simulink model "DemoControlSys"  (R2022b)
settings: Solver=VariableStepAuto  StartTime=0.0  StopTime=10.0  RelTol=1e-3
undefined symbols (not defined in the file): k, ka, kd, ki, kp, kpos, kv
settings Model: Creator=Ilya_Andriyanov  LastModifiedBy=Ilya_Andriyanov

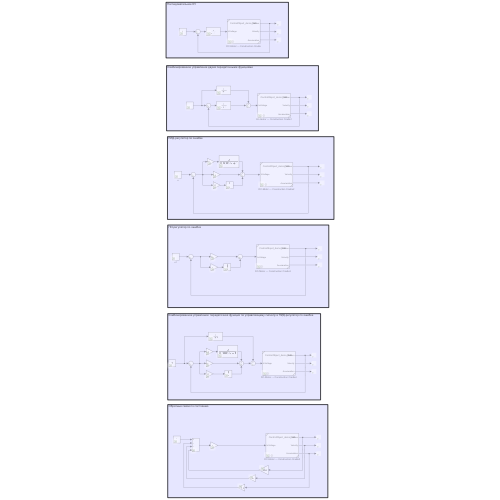
[thumbnail: Simulink's stored preview of the top-level diagram]
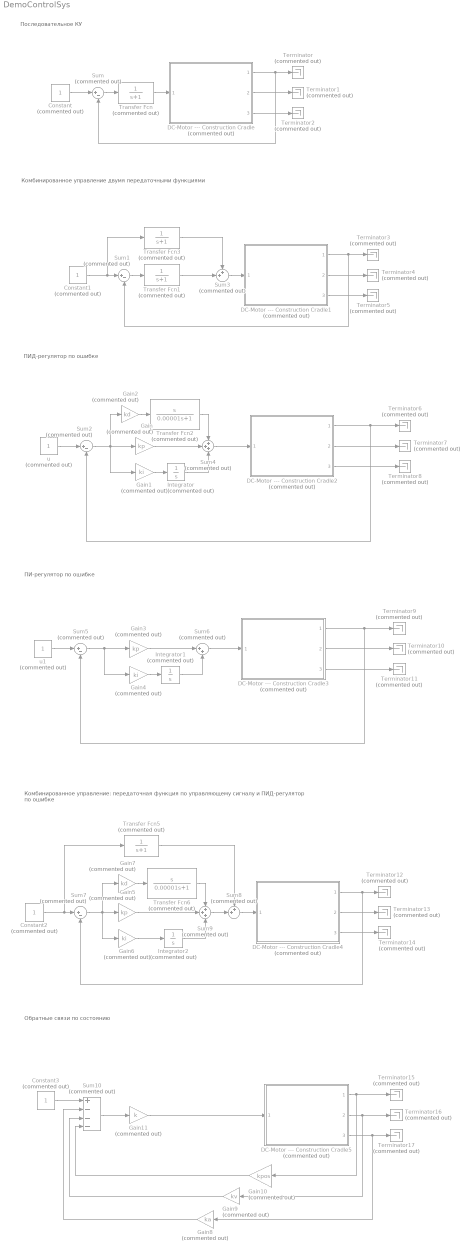
== system DemoControlSys ==
  note: Обратные связи по состоянию
  note: Комбинированное управление: передаточная функция по управляющему сигналу и ПИД-регулятор по ошибке
  note: ПИ-регулятор по ошибке
  note: ПИД-регулятор по ошибке
  note: Комбинированное управление двумя передаточными функциями
  note: Последовательное КУ
  Constant{,1..3} (4 alike) : Constant  Commented=on
  DC-Motor --- Construction Cradle{,1..5} (6 alike) : Subsystem  Commented=on  ReferencedSubsystem=ControlObject_demo_22b  L=0.1  R=0.2  km=1e-3  kw=0.2  J_motor=1e-6  vis_friction_coef_motor=0.001  i_gear=100  J_gear=0.001  vis_friction_coef_gear=0.001  r_wheel=0.1  J_wheel=5  vis_friction_coef_cradle=0.001  veh_mass=20  alpha=5
  Gain : Gain  Commented=on  Gain=kp
  Gain1 : Gain  Commented=on  Gain=ki
  Gain10 : Gain  Commented=on  Gain=kpos
  Gain11 : Gain  Commented=on  Gain=k
  Gain2 : Gain  Commented=on  Gain=kd
  Gain3 : Gain  Commented=on  Gain=kp
  Gain4 : Gain  Commented=on  Gain=ki
  Gain5 : Gain  Commented=on  Gain=kp
  Gain6 : Gain  Commented=on  Gain=ki
  Gain7 : Gain  Commented=on  Gain=kd
  Gain8 : Gain  Commented=on  Gain=ka
  Gain9 : Gain  Commented=on  Gain=kv
  Integrator : Integrator  Commented=on
  Integrator1 : Integrator  Commented=on
  Integrator2 : Integrator  Commented=on
  Sum{,1..2,5,7} (5 alike) : Sum  Commented=on  Inputs=|+-
  Sum10 : Sum  Commented=on  Inputs=+---
  Sum3 : Sum  Commented=on  Inputs=++|
  Sum4 : Sum  Commented=on  Inputs=+++
  Sum6 : Sum  Commented=on  Inputs=|++
  Sum8 : Sum  Commented=on  Inputs=++|
  Sum9 : Sum  Commented=on  Inputs=+++
  Terminator{,1..17} (18 alike) : Terminator  Commented=on
  Transfer Fcn{,1,3,5} (4 alike) : TransferFcn  Commented=on  Denominator=[1 1]
  Transfer Fcn2 : TransferFcn  Commented=on  Numerator=[1 0]  Denominator=[0.00001 1]
  Transfer Fcn6 : TransferFcn  Commented=on  Numerator=[1 0]  Denominator=[0.00001 1]
  u : Constant  Commented=on
  u1 : Constant  Commented=on
  wires:
  DC-Motor --- Construction Cradle/1 -> Sum/2, Terminator/1
  DC-Motor --- Construction Cradle/2 -> Terminator1/1
  DC-Motor --- Construction Cradle/3 -> Terminator2/1
  Sum/1 -> Transfer Fcn/1
  Constant/1 -> Sum/1
  Transfer Fcn/1 -> DC-Motor --- Construction Cradle/1
  Constant1/1 -> Transfer Fcn3/1, Sum1/1
  DC-Motor --- Construction Cradle1/3 -> Terminator5/1
  DC-Motor --- Construction Cradle1/2 -> Terminator4/1
  DC-Motor --- Construction Cradle1/1 -> Terminator3/1, Sum1/2
  DC-Motor --- Construction Cradle2/1 -> Terminator6/1, Sum2/2
  DC-Motor --- Construction Cradle2/2 -> Terminator7/1
  DC-Motor --- Construction Cradle2/3 -> Terminator8/1
  u/1 -> Sum2/1
  Sum3/1 -> DC-Motor --- Construction Cradle1/1
  Sum1/1 -> Transfer Fcn1/1
  Transfer Fcn1/1 -> Sum3/2
  Transfer Fcn3/1 -> Sum3/1
  Gain1/1 -> Integrator/1
  Sum4/1 -> DC-Motor --- Construction Cradle2/1
  Integrator/1 -> Sum4/3
  Gain/1 -> Sum4/2
  Sum2/1 -> Gain2/1, Gain1/1, Gain/1
  Transfer Fcn2/1 -> Sum4/1
  Gain2/1 -> Transfer Fcn2/1
  Sum5/1 -> Gain3/1, Gain4/1
  Sum6/1 -> DC-Motor --- Construction Cradle3/1
  Gain4/1 -> Integrator1/1
  u1/1 -> Sum5/1
  DC-Motor --- Construction Cradle3/3 -> Terminator11/1
  DC-Motor --- Construction Cradle3/2 -> Terminator10/1
  DC-Motor --- Construction Cradle3/1 -> Sum5/2, Terminator9/1
  Integrator1/1 -> Sum6/2
  Gain3/1 -> Sum6/1
  Transfer Fcn5/1 -> Sum8/1
  Sum8/1 -> DC-Motor --- Construction Cradle4/1
  DC-Motor --- Construction Cradle4/1 -> Terminator12/1, Sum7/2
  DC-Motor --- Construction Cradle4/2 -> Terminator13/1
  DC-Motor --- Construction Cradle4/3 -> Terminator14/1
  Constant2/1 -> Sum7/1, Transfer Fcn5/1
  Gain7/1 -> Transfer Fcn6/1
  Transfer Fcn6/1 -> Sum9/1
  Sum7/1 -> Gain7/1, Gain5/1, Gain6/1
  Gain5/1 -> Sum9/2
  Integrator2/1 -> Sum9/3
  Gain6/1 -> Integrator2/1
  Sum9/1 -> Sum8/2
  Constant3/1 -> Sum10/1
  DC-Motor --- Construction Cradle5/3 -> Gain8/1, Terminator17/1
  DC-Motor --- Construction Cradle5/2 -> Gain9/1, Terminator16/1
  DC-Motor --- Construction Cradle5/1 -> Gain10/1, Terminator15/1
  Gain10/1 -> Sum10/4
  Gain9/1 -> Sum10/3
  Gain8/1 -> Sum10/2
  Sum10/1 -> Gain11/1
  Gain11/1 -> DC-Motor --- Construction Cradle5/1
